simulink model "Model"  (R2017b)
settings: Solver=VariableStepAuto  StartTime=0.0  StopTime=10.0  RelTol=1e-3
undefined symbols (not defined in the file): add
settings Model: Creator=aarrieta  LastModifiedBy=aarrieta

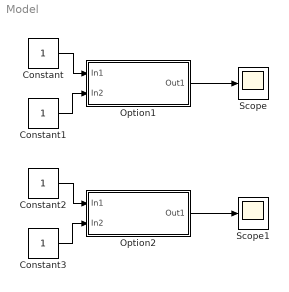
== system Model ==
  Constant{,1..3} (4 alike) : Constant
  Option1 : Subsystem
  Option2 : Subsystem
  Scope : Scope
  Scope1 : Scope
  wires:
  Constant/1 -> Option1/1(In1)
  Constant1/1 -> Option1/2(In2)
  Option1/1(Out1) -> Scope/1
  Option2/1(Out1) -> Scope1/1
  Constant3/1 -> Option2/2(In2)
  Constant2/1 -> Option2/1(In1)

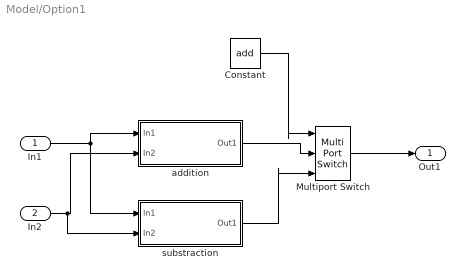
== system Model/Option1 ==
  In1 : Inport
  In2 : Inport  Port=2
  Constant : Constant  Value=add
  Multiport Switch : MultiPortSwitch  Inputs=2
  addition : Subsystem
  substraction : Subsystem
  Out1 : Outport
  wires:
  In1/1 -> substraction/1(In1), addition/1(In1)
  In2/1 -> substraction/2(In2), addition/2(In2)
  addition/1(Out1) -> Multiport Switch/2
  substraction/1(Out1) -> Multiport Switch/3
  Multiport Switch/1 -> Out1/1
  Constant/1 -> Multiport Switch/1

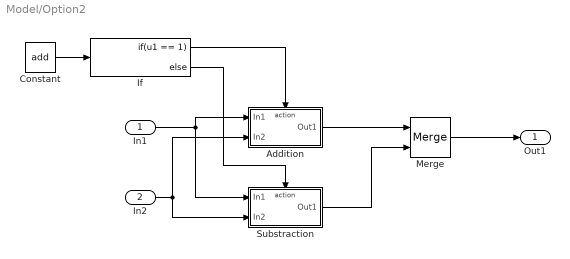
== system Model/Option2 ==
  In1 : Inport
  In2 : Inport  Port=2
  Addition : Subsystem  TreatAsAtomicUnit=on
  Constant : Constant  Value=add
  If : If  IfExpression=u1 == 1
  Merge : Merge
  Substraction : Subsystem  TreatAsAtomicUnit=on
  Out1 : Outport
  wires:
  Constant/1 -> If/1
  Merge/1 -> Out1/1
  Substraction/1(Out1) -> Merge/2
  Addition/1(Out1) -> Merge/1
  In2/1 -> Substraction/2(In2), Addition/2(In2)
  In1/1 -> Substraction/1(In1), Addition/1(In1)
  If/1 -> Addition/Action
  If/2 -> Substraction/Action

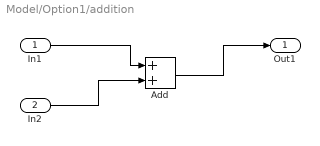
== system Model/Option1/addition ==
  In1 : Inport
  In2 : Inport  Port=2
  Add : Sum
  Out1 : Outport
  wires:
  In1/1 -> Add/1
  In2/1 -> Add/2
  Add/1 -> Out1/1

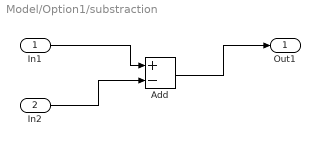
== system Model/Option1/substraction ==
  In1 : Inport
  In2 : Inport  Port=2
  Add : Sum  Inputs=+-
  Out1 : Outport
  wires:
  Add/1 -> Out1/1
  In2/1 -> Add/2
  In1/1 -> Add/1

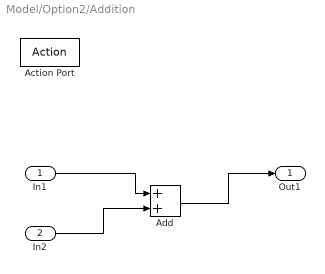
== system Model/Option2/Addition ==
  In1 : Inport
  In2 : Inport  Port=2
  Action Port : ActionPort  ActionType=then
  Add : Sum
  Out1 : Outport
  wires:
  Add/1 -> Out1/1
  In2/1 -> Add/2
  In1/1 -> Add/1

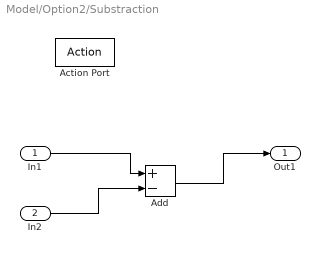
== system Model/Option2/Substraction ==
  In1 : Inport
  In2 : Inport  Port=2
  Action Port : ActionPort  ActionType=else
  Add : Sum  Inputs=+-
  Out1 : Outport
  wires:
  Add/1 -> Out1/1
  In2/1 -> Add/2
  In1/1 -> Add/1
